simulink model "MIMO"  (R2020b)
settings: Solver=VariableStepAuto  StartTime=0.0  StopTime=1.6  RelTol=1e-3
undefined symbols (not defined in the file): A_mimo, B_mimo, D_mimo, H_mimo, KE_mimo, KF_mimo, Kr_mimo, Ts
libraries: cstblocks x2
settings Model: Creator=LACER_GMG  LastModifiedBy=GMG

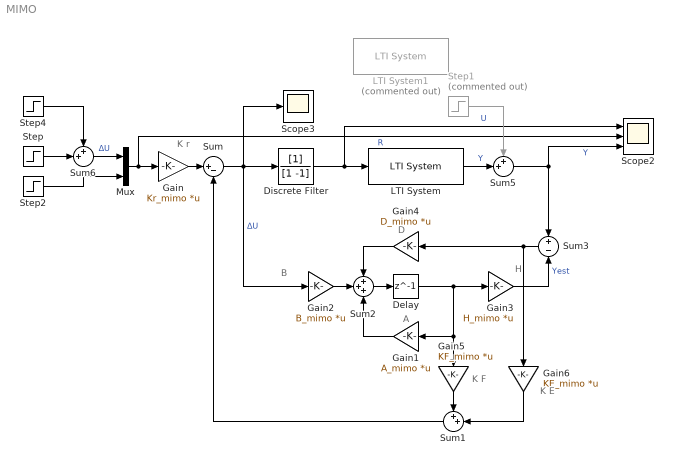
== system MIMO ==
  note: D
  note: A
  note: B
  note: K F
  note: K E
  note: H
  note: K r
  Delay : Delay  DelayLength=1  InitialCondition=[0 0 0 0 0 0]  SampleTime=Ts
  Discrete Filter : DiscreteFilter  Denominator=[1 -1]  FilterStructure=Direct form I  SampleTime=Ts
  Gain : Gain  Gain=Kr_mimo  Multiplication=Matrix(K*u) (u vector)
  Gain1 : Gain  Gain=A_mimo  Multiplication=Matrix(K*u) (u vector)
  Gain2 : Gain  Gain=B_mimo  Multiplication=Matrix(K*u) (u vector)
  Gain3 : Gain  Gain=H_mimo  Multiplication=Matrix(K*u) (u vector)
  Gain4 : Gain  Gain=D_mimo  Multiplication=Matrix(K*u) (u vector)
  Gain5 : Gain  Gain=KF_mimo  Multiplication=Matrix(K*u) (u vector)
  Gain6 : Gain  Gain=KE_mimo  Multiplication=Matrix(K*u) (u vector)
  LTI System : cstblocks/LTI System  sys=Y_mimo  IC=[]
  LTI System1 : cstblocks/LTI System  Commented=on  sys=Integrador  IC=[]
  Mux : Mux  Inputs=2
  Scope2 : Scope  NumInputPorts=3
  Scope3 : Scope
  Step : Step  Time=0.1  After=0.5  SampleTime=Ts
  Step1 : Step  Commented=on  Time=3  SampleTime=Ts
  Step2 : Step  Time=0.1  After=0.3  SampleTime=Ts
  Step4 : Step  After=-0.1  SampleTime=Ts
  Sum : Sum  Inputs=|+-
  Sum1 : Sum  Inputs=++|
  Sum2 : Sum  Inputs=+++
  Sum3 : Sum  Inputs=+|-
  Sum5 : Sum  Inputs=++|
  Sum6 : Sum  Inputs=++|
  wires:
  Gain2/1 -> Sum2/2
  Sum3/1 -> Gain4/1, Gain6/1
  Gain3/1 -> Sum3/2  "Yest"
  Delay/1 -> Gain5/1, Gain1/1, Gain3/1
  Sum2/1 -> Delay/1
  Gain1/1 -> Sum2/3
  Gain5/1 -> Sum1/1
  Gain6/1 -> Sum1/2
  Gain/1 -> Sum/1
  Sum/1 -> Scope3/1, Discrete Filter/1, Gain2/1  "ΔU"
  Sum5/1 -> Scope2/3, Sum3/1  "Y"
  Step/1 -> Sum6/2
  Step2/1 -> Mux/2
  Mux/1 -> Scope2/2, Gain/1  "R"
  Sum1/1 -> Sum/2
  Gain4/1 -> Sum2/1
  Sum6/1 -> Mux/1  "ΔU"
  Step4/1 -> Sum6/1
  Discrete Filter/1 -> Scope2/1, LTI System/1  "U"
  Step1/1 -> Sum5/1
  LTI System/1 -> Sum5/2  "Y"
